simulink model "NCML_first_project"  (R2015a)
settings: Solver=ode4  SolverMode=MultiTasking  StartTime=0.0  StopTime=inf  FixedStep=BKIN_STEP_TIME  RelTol=1e-3
StartFcn:
  |  warndlg('Dexterit-E models cannot run under simulation. Please compile your model and run it from within Dexterit-E.');set_param(bdroot,'SimulationCommand','stop')
model workspace (MAT data in the model file):
  col_x = 1
  col_y = 2
  COLOR_INIT = 6
  COLOR_REACH = 7
  START_TARGET = 1
  MAX_REACH_TIME = 9
  DELAY_POST_TRIAL = 11
  E_STAY_CENTER = 2
  BKIN_STEP_TIME = 0.00025
  DELAY_CUE = 12
  E_CUE_ON = 4
  FX = 5
  FY = 6
  RAMP_SLOPE = 7
  RAMP_CONST = 8
  DELAY_PERTURB = 13
  PERTUB_PROB = 6
  LOAD_LEFT_PROB = 14
  COLOR_CUE0 = 11
  COLOR_CUE25 = 8
  COLOR_CUE50 = 9
  COLOR_CUE75 = 10
  TEXT_SCORE = 12
  SCORE_PIC = 17
  SCORE_TEXT = 18
  DELAY_READY_FIXED = 7
  DELAY_READY_RANDOM = 8
  DELAY_TARGET = 10
  ROTATION = 5
  CUE_TARGET = 2
  MINOR_RADIUS = 4
  MAJOR_RADIUS = 3
  XL_END_TARGET = 3
  XS_END_TARGET = 4
  END_SIZE_PROB = 5
  VISC_X = 1
  VORT_X = 2
  VORT_Y = 3
  VISC_Y = 4
  LOAD_CCW = 15
  LOAD_CW = 16
  DELAY_GO = 19
  GO_TEXT = 20
  E_REACH_TARGET = 5
  E_NOT_HOLD = 7
  E_SCORE = 8
  E_MISS = 9
  E_PERTURB_ON = 10
  MAX_RECOVER = 21
  E_LOCATION_ON = 6
  E_TARGET_GO = 3
  MAX_REACT_TIME = 22
  E_MOVE_OUT_SP = 11
  LOWER_REACH_TIME = 23
  UPPER_REACH_TIME = 24
  E_STAY_TARGET = 12
  CONST_MT = 25
  E_TRIAL_FAIL = 13
libraries: Video x7, General x3, KINARM_general x2, KINARM_EP_loads x2, xpcseriallib x1, KINARM_IO x1, simulink x1, commutil2 x1, xpcnilib x1
CloseFcn:
  | rtwprivate ssgencode ModelCloseRequest b2lab2d
settings Model: ModifiedComment=chris -- Wed Feb 16 09:18:30 2005 -- Version 1.1384  ModifiedHistory=Feb 16/05 - Add error repeat, add offset ramp  ExtModeArmWhenConnect=off  ExtModeLogAll=off  Creator=Chris Grebeldinger  LastModifiedBy=User
settings SolverCC: EnableConcurrentExecution=on  AutoInsertRateTranBlk=on
settings DataIOCC: LimitDataPoints=off  SignalLoggingSaveFormat=ModelDataLogs  SaveOutput=off  SaveTime=off  SignalLoggingName=sigsOut
settings OptimizationCC: BlockReduction=off  BooleanDataType=off  OptimizeBlockIOStorage=off  BufferReuse=off  GlobalBufferReuse=off  ExpressionFolding=off  ExpressionDepthLimit=2147483647  LocalBlockOutputs=off  InitFltsAndDblsToZero=on
settings DebuggingCC: SaveWithParameterizedLinksMsg=none  UnderspecifiedInitializationDetection=Classic  MergeDetectMultiDrivingBlocksExec=none  SignalResolutionControl=TryResolveAllWithWarning  MultiTaskDSMMsg=warning  FcnCallInpInsideContextMsg=UseLocalSettings  StateNameClashWarn=warning  StrictBusMsg=ErrorOnBusTreatedAsVector
settings HardwareCC: ProdIntDivRoundTo=Zero  ProdEndianess=LittleEndian  ProdLongLongMode=on  ProdHWDeviceType=Generic->32-bit x86 compatible  TargetHWDeviceType=32-bit Generic
settings SFSimCC: SimCustomHeaderCode="#include \"stdlib.h\""  SFSimEcho=off  SimParseCustomCode=off
settings RTWCC: SystemTargetFile=slrt.tlc  TemplateMakefile=slrt_default_tmf  Description=Simulink Real-Time  CustomSourceCode="#include \"stdlib.h\""
settings CodeAppCC: MaxIdLength=63
settings SimulinkRealTimeCC: TargetFcnLib=ansi_tfl_tmw.mat  GeneratePreprocessorConditionals=Disable all  xPCisDownloadable=off  xPCisDefaultEnv=off

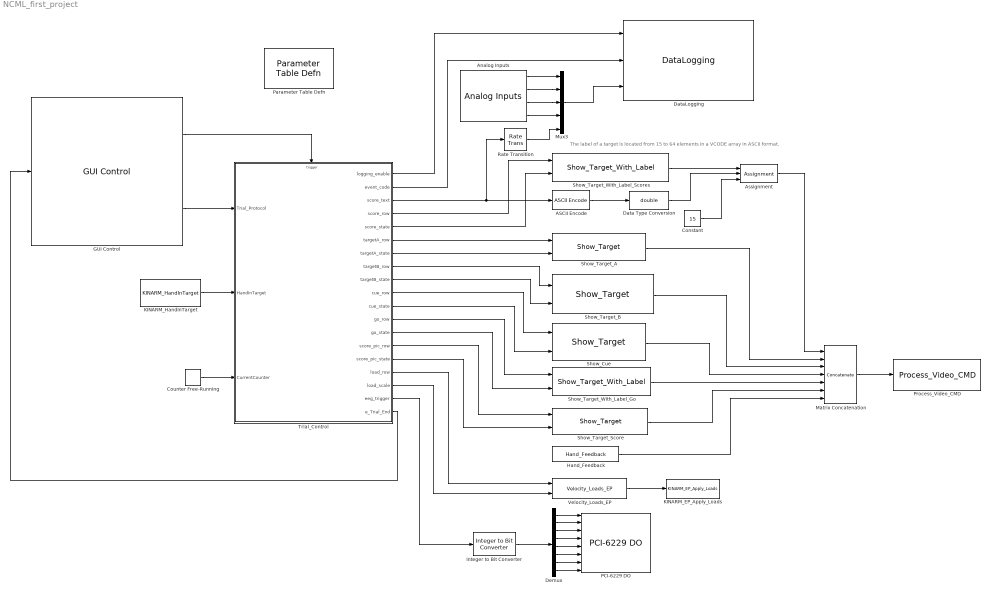
== system NCML_first_project ==
  note: The label of a target is located from 15 to 64 elements in a VCODE array in ASCII format.
  "ASCII Encode " : xpcseriallib/ASCII Encode   format=%d  nvars=1  maxlength=48  vartypes={ 'double' }
  Analog Inputs : KINARM_IO/Analog Inputs  channel=[1:4]  range=[10 10 10 10]  coupling=[0 0 0 0]  scantime6071e=1.28e-5  scantime6229=5e-6  sampletime=0.001  slot=-1  oscantime6071e=0
  Assignment : Assignment  DiagnosticForDimensions=Warning  IndexOptions=Starting index (port)
  Constant : Constant  Value=15  OutDataTypeStr=uint8
  Counter Free-Running : simulink/Sources/Counter Free-Running  NumBits=16  tsamp=0.001
  Data Type Conversion : DataTypeConversion  OutDataTypeStr=double
  DataLogging : General/DataLogging  log_event_codes=on  log_analog_inputs=on
      link override Poll KINARM/EPTorqueCMD: GotoTag=KINARMEPTorqueCMD
      link override Poll KINARM/TorqueCMD: GotoTag=KINARMTorqueCMD
  Demux : Demux  Outputs=8
  GUI Control : General/GUI Control  target_type_str=Circle  Target_Type=1  XYcols=[1 2]  Vcols=3  Lcols=4  indices_padding=[0 0 0 0;0 0 0 0]  task_version=1.0  show_repeat_trial_flag=off
  Hand_Feedback : KINARM_general/Hand_Feedback  feedback_cntl_src=none
  Integer to Bit Converter : commutil2/Integer to Bit Converter  nbits=8  signedInputValues=Unsigned  bitOrder=LSB first  outDtype=Inherit via internal rule
  KINARM_EP_Apply_Loads : KINARM_EP_loads/KINARM_EP_Apply_Loads  up_duration=1500  down_duration=1500  max_force=60
  KINARM_HandInTarget : KINARM_general/KINARM_HandInTarget  use_dominant_hand=on  target_type=Ellipse  num_states=1  attribcol1=[3 4 5]  attribcol2=[4 0 0]  attribcol3=[5 0 0]  attribcol4=[6 0 0]  attribcol5=[0 0 0]
  Matrix Concatenation : Concatenate  NumInputs=7  Mode=Multidimensional array
  Mux3 : Mux  Inputs=5
  PCI-6229 DO : xpcnilib/Digital Output/M Series/PCI-6229 DO  channel=[9,10,11,12,13,14,15,16]  reset=[1]  initValue=[0]  sampletime=0.00025  slot=-1
  Parameter Table Defn : General/Parameter Table Defn  ShowInLibBrowser=0
  Process_Video_CMD : Video/Process_Video_CMD
  Rate Transition : RateTransition
  Show_Cue : Video/Show_Target  target_type=Ellipse  num_states=4  attribcol1=[8 0 0 3 3 5]  attribcol2=[9 0 0 3 3 5]  attribcol3=[10 0 0 3 3 5]  attribcol4=[11 0 0 3 3 5]  attribcol5=[ 0 0 0 0 0 0]  stateindices_padding=[0 0 0 0 0;0 0 0 0 0;0 0 0 0 0;0 0 0 0 0;0 0 0 0 0]  source=dialog  opacity=100  target_display=Both subject and operator displays  num_col=6
  Show_Target_A : Video/Show_Target  target_type=Circle  num_states=2  attribcol1=[6 0 0 3]  attribcol2=[7 0 0 3]  attribcol3=[7 0 0 3]  attribcol4=[0 0 0 0]  attribcol5=[0 0 24 0]  stateindices_padding=[0 0 0 0 0 0 0;0 0 0 0 0 0 0;0 0 0 0 0 0 0;0 0 0 0 0 0 0;0 0 0 0 0 0 0]  source=dialog  opacity=100  target_display=Both subject and operator displays  num_col=4
  Show_Target_B : Video/Show_Target  target_type=Ellipse  num_states=4  attribcol1=[6 0 0 3 4 5]  attribcol2=[7 0 0 3 4 5]  attribcol3=[0 6 -1 3 4 5]  attribcol4=[8 0 0 3 4 5]  attribcol5=[9 0 0 12 0 0]  stateindices_padding=[0 0 0 0 0;0 0 0 0 0;0 0 0 0 0;0 0 0 0 0;0 0 0 0 0]  source=dialog  opacity=100  target_display=Both subject and operator displays  num_col=6
  Show_Target_Score : Video/Show_Target  target_type=Circle  num_states=2  attribcol1=[6 0 0 3]  attribcol2=[7 0 0 3]  attribcol3=[0 0 0 0]  attribcol4=[0 0 0 0]  attribcol5=[0 0 24 0]  stateindices_padding=[0 0 0 0 0 0 0;0 0 0 0 0 0 0;0 0 0 0 0 0 0;0 0 0 0 0 0 0;0 0 0 0 0 0 0]  source=dialog  opacity=100  target_display=Both subject and operator displays  num_col=4
  Show_Target_With_Label_Go : Video/Show_Target_With_Label  target_type=Circle  num_states=1  attribcol1=[0 0 0 0 12 7 3]  attribcol2=[0 0 0 0 13 7 3]  attribcol3=[0 0 0 0 0 0 0]  attribcol4=[0 0 0 0 0 0 0]  attribcol5=[0 0 24 0 0 0 0]  stateindices_padding=[0 0 0 0;0 0 0 0;0 0 0 0;0 0 0 0;0 0 0 0]  source=dialog  opacity=100  target_display=Both subject and operator displays
  Show_Target_With_Label_Scores : Video/Show_Target_With_Label  target_type=Circle  num_states=2  attribcol1=[0 0 0 0 0 6 3]  attribcol2=[0 0 0 0 0 7 3]  attribcol3=[0 0 0 0 0 0 0]  attribcol4=[0 0 0 0 0 0 0]  attribcol5=[0 0 24 0 0 0 0]  stateindices_padding=[0 0 0 0;0 0 0 0;0 0 0 0;0 0 0 0;0 0 0 0]  source=dialog  opacity=100  target_display=Both subject and operator displays
  Trial_Control : Stateflow chart  TreatAsAtomicUnit=on
  Velocity_Loads_EP : KINARM_EP_loads/Velocity_Loads_EP  use_dom_hand=on  loadcol=[1 2 3 4]  source=port  scaling=1  stability=on
  wires:
  KINARM_HandInTarget/1 -> Trial_Control/2(HandInTarget)
  GUI Control/2 -> Trial_Control/1(Trial_Protocol)
  Trial_Control/19(e_Trial_End) -> GUI Control/1
  GUI Control/1 -> Trial_Control/Trigger
  Trial_Control/7(targetA_state) -> Show_Target_A/2
  Trial_Control/6(targetA_row) -> Show_Target_A/1
  Matrix Concatenation/1 -> Process_Video_CMD/1
  Hand_Feedback/1 -> Matrix Concatenation/7
  Show_Target_B/1 -> Matrix Concatenation/3
  Trial_Control/8(targetB_row) -> Show_Target_B/1
  Trial_Control/9(targetB_state) -> Show_Target_B/2
  Trial_Control/16(load_row) -> Velocity_Loads_EP/1
  Analog Inputs/1 -> Mux3/1
  Trial_Control/1(logging_enable) -> DataLogging/1
  Trial_Control/2(event_code) -> DataLogging/2
  Analog Inputs/2 -> Mux3/2
  Analog Inputs/3 -> Mux3/3
  Show_Target_A/1 -> Matrix Concatenation/2
  Velocity_Loads_EP/1 -> KINARM_EP_Apply_Loads/1
  Trial_Control/4(score_row) -> Show_Target_With_Label_Scores/1
  Trial_Control/5(score_state) -> Show_Target_With_Label_Scores/2
  "ASCII Encode "/1 -> Data Type Conversion/1
  Constant/1 -> Assignment/3
  Show_Target_With_Label_Scores/1 -> Assignment/1
  Data Type Conversion/1 -> Assignment/2
  Assignment/1 -> Matrix Concatenation/1
  Trial_Control/3(score_text) -> "ASCII Encode "/1, Rate Transition/1
  Show_Target_Score/1 -> Matrix Concatenation/6
  Trial_Control/14(score_pic_row) -> Show_Target_Score/1
  Trial_Control/15(score_pic_state) -> Show_Target_Score/2
  Trial_Control/10(cue_row) -> Show_Cue/1
  Trial_Control/11(cue_state) -> Show_Cue/2
  Show_Cue/1 -> Matrix Concatenation/4
  Trial_Control/17(load_scale) -> Velocity_Loads_EP/2
  Show_Target_With_Label_Go/1 -> Matrix Concatenation/5
  Trial_Control/13(go_state) -> Show_Target_With_Label_Go/2
  Trial_Control/12(go_row) -> Show_Target_With_Label_Go/1
  Counter Free-Running/1 -> Trial_Control/3(CurrentCounter)
  Trial_Control/18(eeg_trigger) -> Integer to Bit Converter/1
  Demux/1 -> PCI-6229 DO/1
  Demux/2 -> PCI-6229 DO/2
  Demux/3 -> PCI-6229 DO/3
  Demux/4 -> PCI-6229 DO/4
  Demux/5 -> PCI-6229 DO/5
  Demux/6 -> PCI-6229 DO/6
  Demux/7 -> PCI-6229 DO/7
  Demux/8 -> PCI-6229 DO/8
  Integer to Bit Converter/1 -> Demux/1
  Mux3/1 -> DataLogging/3
  Rate Transition/1 -> Mux3/5
  Analog Inputs/4 -> Mux3/4

== stateflow chart NCML_first_project/Trial_Control ==
  settings: sampleTime=0.001
  state Initialize/
    // Both the targets and data logging are initially off.
    targetA_state = 0;
    cue_state = 0;
    go_state = 0;
    targetB_state = 0;
    logging_enable = 0;
    perturb = 0;
    load_scale = 0;
    score_state = 0;
    score_text = 1000;
    score_pic_state = 0;
  state MainTrial
    state ShowFirstTarget/
      // Turn on first target, set loading conditions, enable data logging, and wait for a specified time or until the hand is in the target.
      targetA_row = Trial_Protocol[START_TARGET];
      cue_row = Trial_Protocol[CUE_TARGET];
      go_row = Trial_Protocol[GO_TEXT];
      perturb_prob = Trial_Protocol[PERTUB_PROB]; // Get perturbation probability
      score_pic_row = Trial_Protocol[SCORE_PIC];
      score_row = Trial_Protocol[SCORE_TEXT];
      targetA_state = 1;
      cue_state = 0;
      go_state = 0;
      targetB_state = 0;
      logging_enable = 0;
      event_code = 0;
    state StayAtFirstTarget/
      // Log an event that target was reached, begin data logging, change the first target's state, and then wait for a specified time.
      // The wait time may have both a fixed and a random component. The hand must stay in the target for the full wait time.
      logging_enable = 1;
      event_code = E_STAY_CENTER;
      targetA_state = 2;
      tickCount = Trial_Protocol[DELAY_READY_FIXED] + Trial_Protocol[DELAY_READY_RANDOM] * rand() / RAND_MAX;
      perturb_random = 100 * rand() / RAND_MAX; // Generate a random number for determining perturbation
      score_state = 0;
      score_pic_state = 0;
      targetB_row = Trial_Protocol[XL_END_TARGET];
    state ShowTargetWithCueWhileStayAtTargetA/
      // Turn on second target with cue and log an event indicating this has occurred. Then wait until a specified time has elapsed.
      event_code = E_CUE_ON;
      tickCount = Trial_Protocol[DELAY_CUE];
      size_prob = Trial_Protocol[END_SIZE_PROB];
      size_random = 100 * rand() / RAND_MAX; // Generate a random number for determining target size
    state ShowTargetLocationWhileStayAtTargetA/
      // Show target B location after cue
      event_code = E_LOCATION_ON;
      tickCount = Trial_Protocol[DELAY_GO];
      cue_state = 0;
      targetB_state = 3;
      load_prob = Trial_Protocol[LOAD_LEFT_PROB];
      load_random = 100 * rand() / RAND_MAX; // Generate a random number for determining perturbation direction
    state ShowSecondTarget/
      // Turn on second target and log an event indicating this has occurred. Then wait until the hand is the target or until a specified time has elapsed.
      event_code = E_TARGET_GO;
      // Put GO cue here +++++++++++++++++++++++++++++++++++++++++++++++++//
      go_state = 1;
      targetB_state = 1;
      tickCount = Trial_Protocol[MAX_REACT_TIME];
    state OnceMoveOutFirstTarget/
      // Once the hand moved out of the first target
      en: tickMoveOnset = CurrentCounter;
      event_code = E_MOVE_OUT_SP;
      go_state = 0;
      targetA_state = 0;
      tickCount = Trial_Protocol[MAX_REACH_TIME];
      ex: tickElapsed = temporalCount(msec);
    state DelayPerturb/ [commented out]
      // delay a period before applying pertub
      tickCount_perturb = Trial_Protocol[DELAY_PERTURB];
      tickCount = tickCount - tickElapsed;
      du: tickElapsed = temporalCount(msec);
    state Perturb/
      event_code = E_PERTURB_ON;
      load_scale = 1;
      tickCount = tickCount - tickElapsed;
    state ReachSecondTarget/
      // Log an event that the second target was reached
      en: tickMove = CurrentCounter - tickMoveOnset;
      event_code = E_REACH_TARGET;
      tickElapsed = 0;
    state StayAtSecondTarget/
      // Log an event that specific time to stay at the second target was reached.
      event_code = E_STAY_TARGET;
      tickCount = Trial_Protocol[DELAY_TARGET];
      tickCount = tickCount - tickElapsed;
    state NotStayAtTarget/
      event_code = E_NOT_HOLD;
      targetB_state = 1;
      tickCount = Trial_Protocol[MAX_RECOVER];
      ex: tickElapsed = temporalCount(msec);
    state Score/
      // Get point
      event_code = E_SCORE;
      score_text = score_text + 1;
      targetB_state = 0;
      score_pic_state = 2;
      score_state = 2;
    state Miss/
      // Fail
      event_code = E_MISS;
      targetB_state = 0;
      score_pic_state = 1;
      score_state = 1;
      go_state = 0;
    state EndOfTrial/
      // Set the post-trial delay.
      tickCount = Trial_Protocol[DELAY_POST_TRIAL];
    ShowFirstTarget -> StayAtFirstTarget : [HandInTarget[targetA_row] == 1]
    (junction 155) -> ShowFirstTarget
    StayAtFirstTarget -> (junction 155) [order 2] : [HandInTarget[targetA_row] == 0]
    StayAtFirstTarget -> (junction 106) [order 1] : after(tickCount, msec)
    (junction 106) -> (junction 109) [order 1] : [perturb_prob == 75]
    (junction 106) -> (junction 107) [order 2]
    (junction 109) -> (junction 111) : {cue_state = 3;}
    (junction 107) -> (junction 113) [order 1] : [perturb_prob == 50]
    (junction 107) -> (junction 118) [order 2] : {cue_state = 1;}
    (junction 113) -> (junction 115) : {cue_state = 2;}
    (junction 118) -> (junction 121) [order 1] : [perturb_random >= perturb_prob]
    (junction 115) -> (junction 118)
    (junction 111) -> (junction 115)
    (junction 121) -> (junction 126) : {perturb = 0;}
    (junction 118) -> (junction 127) [order 2] : {perturb = 1;}
    (junction 127) -> (junction 126)
    (junction 126) -> ShowTargetWithCueWhileStayAtTargetA
    ShowTargetWithCueWhileStayAtTargetA -> ShowTargetLocationWhileStayAtTargetA [order 1] : after(tickCount, msec)
    ShowTargetWithCueWhileStayAtTargetA -> (junction 213) [order 2] : [HandInTarget[targetA_row] == 0]
    ShowTargetLocationWhileStayAtTargetA -> (junction 213) [order 2] : [HandInTarget[targetA_row] == 0]
    (junction 213) -> (junction 236)
    ShowTargetLocationWhileStayAtTargetA -> (junction 291) [order 1] : after(tickCount, msec)
    (junction 291) -> (junction 295) [order 1] : [size_random > size_prob]
    (junction 295) -> (junction 294) : {targetB_row = Trial_Protocol[XS_END_TARGET];}
    (junction 291) -> (junction 292) [order 2]
    (junction 294) -> (junction 292)
    (junction 292) -> (junction 134)
    (junction 134) -> (junction 202) [order 1] : [load_random > load_prob]
    (junction 202) -> (junction 203) : {load_row = Trial_Protocol[LOAD_CW];}
    (junction 134) -> (junction 140) [order 2] : {load_row = Trial_Protocol[LOAD_CCW];}
    (junction 203) -> (junction 140)
    (junction 140) -> ShowSecondTarget
    ShowSecondTarget -> OnceMoveOutFirstTarget [order 2] : [HandInTarget[targetA_row] == 0]
    ShowSecondTarget -> (junction 149) [order 1] : after(tickCount, msec)
    OnceMoveOutFirstTarget -> (junction 149) [order 1] : after(tickCount, msec)
    (junction 236) -> (junction 149)
    (junction 149) -> (junction 148)
    OnceMoveOutFirstTarget -> ReachSecondTarget [order 3] : [perturb == 0 && HandInTarget[targetB_row] == 1]
    OnceMoveOutFirstTarget -> DelayPerturb [commented out] : [perturb == 1]
    OnceMoveOutFirstTarget -> Perturb [order 2] : [perturb == 1]
    DelayPerturb -> Perturb [commented out] : after(tickCount_perturb, e_clk)
    Perturb -> (junction 148) [order 1] : after(tickCount, msec)
    (junction 148) -> (junction 152) : {score_text = score_text - 1;}
    Perturb -> ReachSecondTarget [order 2] : [HandInTarget[targetB_row] == 1]
    ReachSecondTarget -> (junction 268)
    (junction 268) -> (junction 247) [order 1] : [ Trial_Protocol[CONST_MT] == 1 && perturb == 0 && (tickMove < Trial_Protocol[LOWER_REACH_TIME] || tickMove > Trial_Protocol[UPPER_REACH_TIME]) ]
    (junction 265) -> (junction 268)
    (junction 247) -> (junction 252) : {targetB_state = 4;}
    (junction 268) -> (junction 251) [order 2] : {targetB_state = 2;}
    NotStayAtTarget -> (junction 265) [order 2] : [HandInTarget[targetB_row] == 1]
    (junction 252) -> (junction 251)
    (junction 251) -> StayAtSecondTarget
    StayAtSecondTarget -> (junction 273) [order 1] : after(tickCount, msec)
    StayAtSecondTarget -> NotStayAtTarget [order 2] : [HandInTarget[targetB_row] == 0]
    NotStayAtTarget -> (junction 152) [order 1] : after(tickCount, msec)
    (junction 152) -> (junction 275)
    (junction 273) -> (junction 275) [order 2]
    (junction 273) -> Score [order 1] : [targetB_state == 2]
    (junction 275) -> Miss
    Score -> (junction 189)
    Miss -> (junction 189) : {event_code = E_TRIAL_FAIL;}
    (junction 189) -> EndOfTrial
  state Inter_Trial_State/
    // Turn off both targets, turn off data logging, reset the
    // event code, and send the e_Trial_End Stateflow event.
    event_code = 0;
    targetA_state = 0;
    cue_state = 0;
    targetB_state = 0;
    logging_enable = 0;
    perturb = 0;
    load_scale = 0;
    e_Trial_End;
  (default) -> Initialize
  Initialize -> ShowFirstTarget
  Inter_Trial_State -> ShowFirstTarget : after(tickCount, msec)
  MainTrial -> Inter_Trial_State : e_ExitTrialNow/
      | tickCount = 1;
  EndOfTrial -> Inter_Trial_State
  data: logging_enable output boolean =0; Trial_Protocol input double; HandInTarget input double; event_code output uint16 [0..] =0; score_text output double; score_row output double; score_state output double; targetA_row output double [1..32]; targetA_state output double =0; targetB_row output double; targetB_state output double =0; cue_row output double; cue_state output double; go_row output double; go_state output double; score_pic_row output double; score_pic_state output double; load_row output double [1..32]; tickCount local double; perturb local boolean; tickElapsed local double; tickCount_perturb local double; perturb_random local double; perturb_prob local double; load_prob local double; load_random local double; size_prob local double; size_random local double; load_scale output double; tickMove local uint16; tickMoveOnset local uint16; CurrentCounter input uint16; eeg_trigger output double
  data targetA_row settings: description=index of the row currently being used in the TargetTable
  data load_row settings: description=current index into the loadtable
  events: e_clk input RISING_EDGE_EVENT; e_ExitTrialNow input EITHER_EDGE_EVENT; e_Trial_End output EITHER_EDGE_EVENT
